simulink model "TIF_avance3"  (R2021b)
settings: Solver=VariableStepAuto  StartTime=0.0  StopTime=10  RelTol=1e-3
undefined symbols (not defined in the file): a11, a13, a23, a31, a33, a42, a44, b, B, J, k1, k10, k11, k2, k3, k4, k5, k6, k7, k8, k9, L1, L2, L3, L4, lamb_ref, Lr, Ls, np, Rpower, Rr, Rs, Rspeed, Rsvolt, TSSimP, Udc
libraries: eeTransforms x2, spsUniversalBridgeLib x1, spsAsynchronousMachineSIUnitsLib x1, spsPWMGeneratorMultilevelLib x1, spsDCVoltageSourceLib x1, spsVoltageMeasurementLib x1, spspowerguiLib x1
settings Model: Creator=Administrador  LastModifiedBy=USER

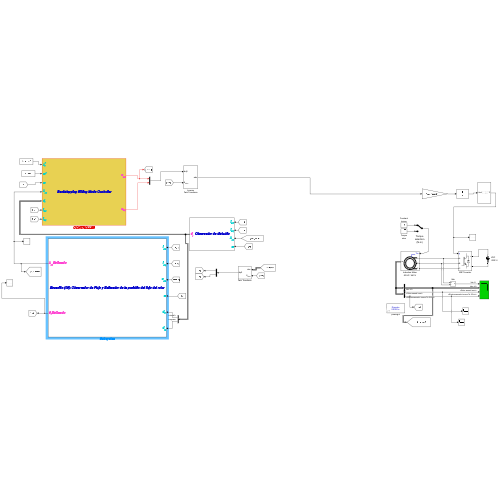
[thumbnail: Simulink's stored preview of the top-level diagram]
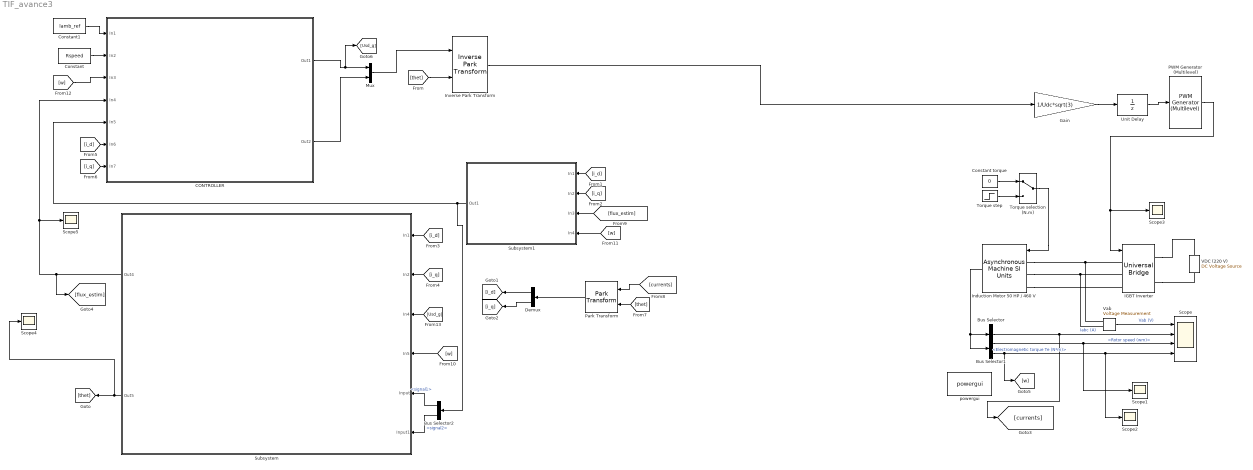
== system TIF_avance3 ==
  Bus Selector : BusSelector  OutputSignals=Stator measurements.Stator current is_a (A),Stator measurements.Stator current is_b (A),Stator measurements.Stator current is_c (A)  OutputAsBus=on
  Bus Selector1 : BusSelector  OutputSignals=Mechanical.Rotor speed (wm),Mechanical.Electromagnetic torque Te (N*m)
  Bus Selector2 : BusSelector  OutputSignals=signal1,signal2
  CONTROLLER : Subsystem
      mask Display:
      | color('magenta'); port_label('output',1,'u_{sd}','texmode', 'on')
      | color('magenta'); port_label('output',2,'u_{sq}','texmode', 'on')
      | color('cyan'); port_label('input',1,'\lambda_r^\ast','texmode', 'on')
      | color('cyan'); port_label('input',2,'\omega^\ast','texmode', 'on')
      | color('cyan'); port_label('input',3,'\omega','texmode', 'on')
      | color('cyan'); port_label('input',4,'\lambda_{rd}','texmode', 'on')
      | color('cyan'); port_label('input',5,'d_{l}','texmode', 'on')
      | color('cyan'); port_label('input',6,'i_{sd}','texmode', 'on')
      | color('cyan'); port_label('input',7,'i_{sq}','texmode', 'on')
      | color('blue'); disp('Backstepping Sliding Mode Controller')
  Constant : Constant  Value=Rspeed
  Constant torque : Constant  Value=0
  Constant1 : Constant  Value=lamb_ref
  Demux : Demux  Outputs=2
  Gain : Gain  Gain=1/Udc*sqrt(3)
  IGBT Inverter : spsUniversalBridgeLib/Universal Bridge  Arms=3  SnubberResistance=1000  SnubberCapacitance=inf  Device=IGBT / Diodes  Ron=1e-3  Lon=0  ForwardVoltages="[  0.8  0.8  ]"  ForwardVoltage=.8  GTOparameters=[ 1e-6 , 1e-6 ]  IGBTparameters=[ 1e-6 , 2e-6 ]  Measurements=None  Measurements_2=None  converterType=Rectifier
      settings: AttributesFormatString=\n
  Induction Motor 50 HP / 460 V : spsAsynchronousMachineSIUnitsLib/Asynchronous Machine SI Units  RotorType=Squirrel-cage  PresetModel=No  MechanicalLoad=Torque Tm  ShowDetailedParameters=on  ReferenceFrame=Stationary  Units=SI  MeasurementBus=off  NominalParameters=[ Rpower, Rsvolt, 60 ]  VoltageRatio=1  Stator=[ Rs Ls ]  Rotor="[ Rr  Lr ]"  Cage1=[ 0.022 0.226/377]  Cage2=[ 0.022 0.226/377]  Lm=Lm  Mechanical="[J  B np ]"  PolePairs=2  InitialConditions="[ 1, 0 ,  0 , 0 , 0 , 0 , 0 , 0 ]"  SimulateSaturation=off  Saturation=[0 0;0 0]  LoadFlowParameters=0  TsPowergui=0  TsBlock=-1  IterativeModel=Trapezoidal non iterative  IterativeDiscreteModel=Trapezoidal non iterative  Pmec=0
      settings: AttributesFormatString=\n
  Inverse Park Transform : eeTransforms/Inverse Park Transform  AxisAlignment=Q-axis  PowerInvariant=off
  Mux : Mux  Inputs=2
  PWM Generator (Multilevel) : spsPWMGeneratorMultilevelLib/PWM Generator (Multilevel)  BridgeType=Half-bridge  NumberOfBridges=3  Fc=10e3  Ts=TSSimP  ShowCarriersOutport=off
      settings: SourceProductBaseCode=PS
  Park Transform : eeTransforms/Park Transform  AxisAlignment=Q-axis  PowerInvariant=off
  Scope : Scope  NumInputPorts=4
  Scope{1..5} (5 alike) : Scope
  Subsystem : Subsystem
      mask Display:
      | color('magenta'); port_label('output',1,'\lambda_{rd}Estimado','texmode', 'on')
      | color('magenta'); port_label('output',2,'\theta_rEstimado','texmode', 'on')
      | color('cyan'); port_label('input',1,'i_{sd}','texmode', 'on')
      | color('cyan'); port_label('input',2,'i_{sq}','texmode', 'on')
      | color('cyan'); port_label('input',3,'u_{sd}','texmode', 'on')
      | color('cyan'); port_label('input',4,' \omega','texmode', 'on')
      | color('cyan'); port_label('input',5,'d_{l1}','texmode', 'on')
      | color('cyan'); port_label('input',6,'d_{l2}','texmode', 'on')
      | 
      | color('blue'); disp('Ecuación (03): Observador de Flujo y Estimador de la posición del flujo del rotor ')
  Subsystem1 : Subsystem
      mask Display:
      | color('magenta'); port_label('output',1,'d_{l}','texmode', 'on')
      | 
      | 
      | color('cyan'); port_label('input',4,'\omega','texmode', 'on')
      | color('cyan'); port_label('input',3,'\lambda_{rd}','texmode', 'on')
      | 
      | color('cyan'); port_label('input',1,'i_{sd}','texmode', 'on')
      | color('cyan'); port_label('input',2,'i_{sq}','texmode', 'on')
      | color('blue'); disp('Observador de disturbio')
  Torque selection (N.m) : ManualSwitch
  Torque step : Step  Time=1.8  After=200  SampleTime=0
  Unit Delay : UnitDelay  SampleTime=TSSimP  HasFrameUpgradeWarning=on
  VDC (220 V) : spsDCVoltageSourceLib/DC Voltage Source  Description=source block  Amplitude=780  Measurements=None
      settings: AttributesFormatString=\n
  Vab : spsVoltageMeasurementLib/Voltage Measurement  Tag=PoWeRsYsTeMmEaSuReMeNt  PhasorSimulation=off  OutputType=Magnitude  PSBequivalent=0
  powergui : spspowerguiLib/powergui  Priority=2  SimulationMode=Discrete  SampleTime=TSSimP  frequency=60  Iterations=50  frequencyindice=60  Pbase=100e6  ErrMax=1e-4  UnitsV=kV  UnitsW=MW  buscounter=0  FunctionMessages=off  echomessages=off  EnableUseOfTLC=off  CurrentSourceSwitches=off  DisableSnubberDevices=off  DisableRonSwitches=off  DisableVfSwitches=off  DisplayEquations=off  AutomaticDiscreteSolvers=off  SolverType=Tustin/Backward Euler (TBE)  Interpol=off  ExternalGateDelay=off  methode=off  Ts=100  x0status=blocks  SPID=off  SwTol=0  HookPort=off  NonlinearTolerance=0  nMaxIteration=15  ContinueOnMaxIteration=off  RestoreLinks=warning  ResistiveCurrentMeasurement=off  Frange=[0:2:500]  Ylog=off  Xlog=on  ShowGrid=off  save=off  variable=ZData  structure=0  ZoomFFT=on  StartTime=0.0  cycles=1  DisplayStyle=off  fundamental=60  FreqAxis=off  MaxFrequency=1000  frequencyindicesteady=1  RmsSteady=1  display=off
  wires:
  Subsystem/1(Out4) -> [flux_estim], CONTROLLER/4(In4), Scope5/1
  Subsystem1/1(Out1) -> Bus Selector2/1, CONTROLLER/5(In5)
  CONTROLLER/1(Out1) -> [Usd_g], Mux/1
  CONTROLLER/2(Out2) -> Mux/2
  Mux/1 -> Inverse Park Transform/1
  Subsystem/2(Out5) -> Scope4/1, [thet]
  [thet] -> Inverse Park Transform/2
  Park Transform/1 -> Demux/1
  Demux/1 -> [i_d]
  Demux/2 -> [i_q]
  [i_q] -> Subsystem1/2(In2)
  [i_d] -> Subsystem1/1(In1)
  [i_q] -> Subsystem/2(In2)
  [i_d] -> Subsystem/1(In1)
  [i_d] -> CONTROLLER/6(In6)
  [i_q] -> CONTROLLER/7(In7)
  [thet] -> Park Transform/2
  PWM Generator (Multilevel)/1 -> Scope3/1, IGBT Inverter/1
  Torque selection (N.m)/1 -> Induction Motor 50 HP / 460 V/1
  Torque step/1 -> Torque selection (N.m)/2
  Bus Selector1/2 -> [w], Scope2/1, Scope/4  "<Electromagnetic torque Te (N*m)>"
  Bus Selector1/1 -> Scope1/1, Scope/3  "<Rotor speed (wm)>"
  Vab/1 -> Scope/1  "Vab (V)"
  Bus Selector/1 -> [currents], Scope/2  "Iabc (A)"
  Gain/1 -> Unit Delay/1
  Unit Delay/1 -> PWM Generator (Multilevel)/1
  Constant torque/1 -> Torque selection (N.m)/1
  Induction Motor 50 HP / 460 V/1 -> Bus Selector1/1, Bus Selector/1
  Inverse Park Transform/1 -> Gain/1
  [currents] -> Park Transform/1
  [flux_estim] -> Subsystem1/3(In3)
  [w] -> Subsystem/4(In5)
  [w] -> Subsystem1/4(In4)
  [w] -> CONTROLLER/3(In3)
  Bus Selector2/1 -> Subsystem/5(Input)  "<signal1>"
  Bus Selector2/2 -> Subsystem/6(Input1)  "<signal2>"
  [Usd_g] -> Subsystem/3(In4)
  Constant/1 -> CONTROLLER/2(In2)
  Constant1/1 -> CONTROLLER/1(In1)
  connections:
  Vab/LConn1 -- Induction Motor 50 HP / 460 V/LConn1 -- IGBT Inverter/LConn1
  Vab/LConn2 -- Induction Motor 50 HP / 460 V/LConn2 -- IGBT Inverter/LConn2
  IGBT Inverter/RConn2 -- VDC (220 V)/LConn1
  IGBT Inverter/RConn1 -- VDC (220 V)/RConn1
  Induction Motor 50 HP / 460 V/LConn3 -- IGBT Inverter/LConn3

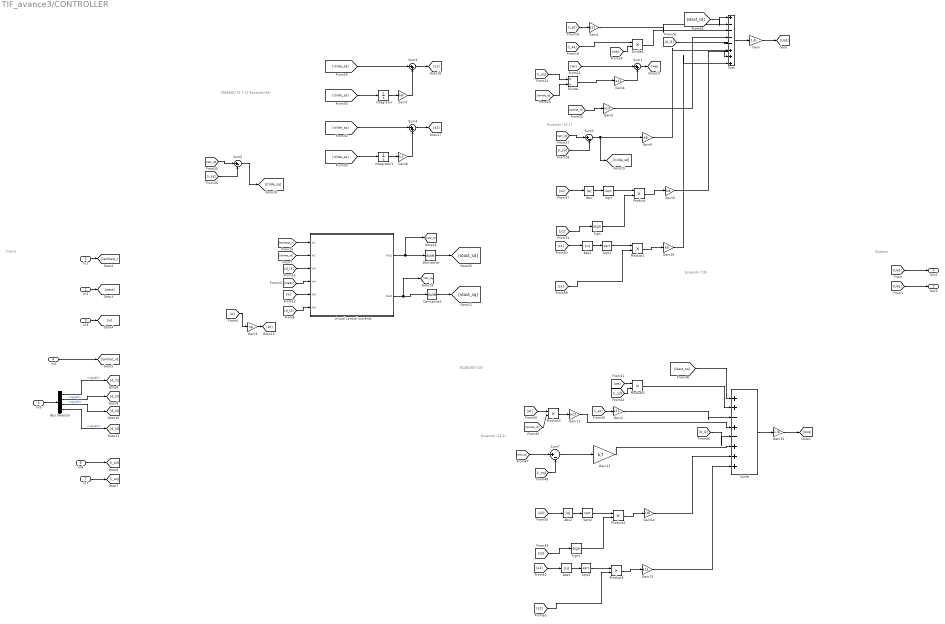
== system TIF_avance3/CONTROLLER ==
  note: ECUACIÓN (20)
  note: Ecuación (15.2)
  note: Ecuación (15.1)
  note: Ecuación (19)
  note: Inputs
  note: Outputs
  note: CREANDO S1 Y S2
      | Ecuación(16)
  In1 : Inport
  In2 : Inport  Port=2
  In3 : Inport  Port=3
  In4 : Inport  Port=4
  In5 : Inport  Port=5
  In6 : Inport  Port=6
  In7 : Inport  Port=7
  Abs{,1..3} (4 alike) : Abs
  Bus Selector : BusSelector  OutputSignals=signal1,signal2,signal3,signal4
  Derivative : Derivative
  Derivative1 : Derivative
  Divide : Product  Inputs=*/
  Divide1 : Product  Inputs=**
  Gain : Gain  Gain=1./b
  Gain1 : Gain  Gain=a11
  Gain10 : Gain  Gain=k9
  Gain11 : Gain  Gain=a23
  Gain12 : Gain  Gain=k7
  Gain13 : Gain  Gain=k11
  Gain14 : Gain  Gain=k10
  Gain15 : Gain  Gain=1./b
  Gain2 : Gain  Gain=a11
  Gain3 : Gain  Gain=np
  Gain4 : Gain  Gain=a31
  Gain5 : Gain  Gain=a13
  Gain6 : Gain  Gain=k6
  Gain7 : Gain  Gain=k6
  Gain8 : Gain  Gain=k7
  Gain9 : Gain  Gain=k8
  Integrator : Integrator
  Integrator1 : Integrator
  Product{,1..5} (6 alike) : Product
  Sign : Signum
  Sign1 : Signum
  Sqrt{,1..3} (4 alike) : Sqrt  SaturateOnIntegerOverflow=on
  Sum : Sum  Inputs=|+|----|+++|
  Sum1 : Sum  Inputs=|++
  Sum2 : Sum  Inputs=|+-
  Sum3 : Sum  Inputs=|++
  Sum4 : Sum  Inputs=|++
  Sum5 : Sum  Inputs=|+-
  Sum6 : Sum  Inputs=|++|-|+|-|+++
  Sum7 : Sum  Inputs=|+-
  "virtual control currents " : Subsystem
      mask Display:
      | color('blue'); port_label('output',1,'i_{sd}^{\ast}','texmode', 'on')
      | color('blue'); port_label('output',2,'i_{sq}^{\ast}','texmode', 'on')
      | color('green'); port_label('input',1,'\lambda_{r}^{\ast}','texmode', 'on')
      | color('green'); port_label('input',2,'\lambda_{rd}','texmode', 'on')
      | color('green'); port_label('input',3,'d_{l3}','texmode', 'on')
      | color('green'); port_label('input',4,'\omega^{\ast}','texmode', 'on')
      | color('green'); port_label('input',5,'\omega','texmode', 'on')
      | color('green'); port_label('input',6,'d_{l4}','texmode', 'on')
      | color('black'); disp(' Ecuación (13)')
  Out1 : Outport
  Out2 : Outport  Port=2
  wires:
  Gain1/1 -> Sum/2
  Sqrt/1 -> Product/1
  In3/1 -> [w]
  In1/1 -> [lambast_r]
  [wr] -> Sum1/1
  "virtual control currents "/2(Out2) -> [iast_sq], Derivative1/1
  [lamhat_rd] -> "virtual control currents "/2(In2)
  [wr] -> Product3/1
  Sum/1 -> Gain/1
  [s1] -> Abs/1
  [lamhat_rd] -> Gain5/1
  [Usq] -> Out2/1
  [itilde_sd] -> Integrator/1
  [w] -> Gain3/1
  Sqrt3/1 -> Product5/1
  In4/1 -> [lamhat_rd]
  Gain4/1 -> Sum1/2
  Integrator1/1 -> Gain8/1
  Abs2/1 -> Sqrt2/1
  [Usd] -> Out1/1
  In2/1 -> [wast]
  Sum6/1 -> Gain15/1
  [d_l4] -> "virtual control currents "/6(In6)
  "virtual control currents "/1(Out1) -> [iast_sd], Derivative/1
  [s2] -> Abs2/1
  Gain/1 -> [Usd]
  [itilde_sq] -> Integrator1/1
  Sum4/1 -> [s2]
  [lambast_r] -> "virtual control currents "/1(In1)
  Gain3/1 -> [wr]
  [s2] -> Abs3/1
  Sum3/1 -> [s1]
  [i_sd] -> Gain1/1
  Abs3/1 -> Sqrt3/1
  [i_sq] -> Divide/1
  Gain14/1 -> Sum6/7
  Divide/1 -> Gain4/1
  Gain13/1 -> Sum6/8
  Product1/1 -> Gain10/1
  [d_l3] -> "virtual control currents "/3(In3)
  [itilde_sq] -> Sum4/1
  Gain5/1 -> Sum/4
  [lamhat_rd] -> Divide/2
  [s1] -> Product1/2
  Sign/1 -> Product/2
  [wast] -> "virtual control currents "/4(In4)
  Product2/1 -> Sum6/2
  Sum1/1 -> [we]
  Derivative1/1 -> [idast_sq]
  Sum2/1 -> Gain6/1, [itilde_sd]
  [w] -> "virtual control currents "/5(In5)
  [d_l1] -> Sum/5
  Integrator/1 -> Gain7/1
  Gain9/1 -> Sum/7
  Gain10/1 -> Sum/8
  Gain8/1 -> Sum4/2
  Gain2/1 -> Sum6/3
  Divide1/1 -> Sum/3
  Product5/1 -> Gain13/1
  [we] -> Divide1/2
  [idast_sq] -> Sum6/1
  [i_sq] -> Divide1/1
  Gain7/1 -> Sum3/2
  [i_sd] -> Sum2/2
  [s2] -> Sign1/1
  Sqrt2/1 -> Product4/1
  Gain15/1 -> [Usq]
  Product4/1 -> Gain14/1
  [s2] -> Product5/2
  Sign1/1 -> Product4/2
  [i_sq] -> Gain2/1
  [lamhat_rd] -> Product3/2
  [itilde_sd] -> Sum3/1
  Gain6/1 -> Sum/6
  Sqrt1/1 -> Product1/1
  Abs/1 -> Sqrt/1
  [idast_sd] -> Sum/1
  Derivative/1 -> [idast_sd]
  [s1] -> Sign/1
  [iast_sq] -> Sum5/1
  [i_sq] -> Sum5/2
  Sum5/1 -> [itilde_sq]
  [we] -> Product2/1
  [iast_sd] -> Sum2/1
  Product/1 -> Gain9/1
  [s1] -> Abs1/1
  Abs1/1 -> Sqrt1/1
  [i_sq] -> Sum7/2
  [i_sd] -> Product2/2
  Gain11/1 -> Sum6/4
  Sum7/1 -> Gain12/1
  Product3/1 -> Gain11/1
  [iast_sq] -> Sum7/1
  Gain12/1 -> Sum6/6
  [d_l2] -> Sum6/5
  In5/1 -> Bus Selector/1
  In7/1 -> [i_sq]
  In6/1 -> [i_sd]
  Bus Selector/1 -> [d_l1]  "<signal1>"
  Bus Selector/2 -> [d_l2]  "<signal2>"
  Bus Selector/3 -> [d_l3]  "<signal3>"
  Bus Selector/4 -> [d_l4]  "<signal4>"

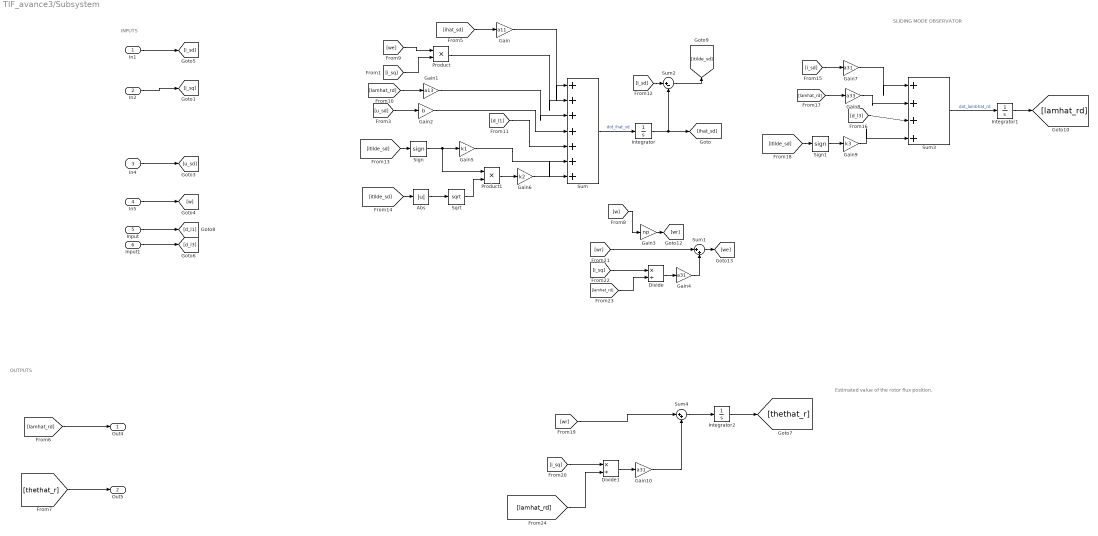
== system TIF_avance3/Subsystem ==
  note: SLIDING MODE OBSERVATOR
  note: OUTPUTS
  note: INPUTS
  note: Estimated value
      | of the rotor flux position.
  In1 : Inport
  In2 : Inport  Port=2
  In4 : Inport  Port=3
  In5 : Inport  Port=4
  Input : Inport  Port=5
  Input1 : Inport  Port=6
  Abs : Abs
  Divide : Product  Inputs=*/
  Divide1 : Product  Inputs=*/
  Gain : Gain  Gain=a11
  Gain1 : Gain  Gain=a13
  Gain10 : Gain  Gain=a31
  Gain2 : Gain  Gain=b
  Gain3 : Gain  Gain=np
  Gain4 : Gain  Gain=a31
  Gain5 : Gain  Gain=k1
  Gain6 : Gain  Gain=k2
  Gain7 : Gain  Gain=a31
  Gain8 : Gain  Gain=a33
  Gain9 : Gain  Gain=k3
  Integrator : Integrator
  Integrator1 : Integrator  InitialCondition=0.2
  Integrator2 : Integrator
  Product : Product
  Product1 : Product
  Sign : Signum
  Sign1 : Signum
  Sqrt : Sqrt  SaturateOnIntegerOverflow=on
  Sum : Sum  Inputs=|+++++++|
  Sum1 : Sum  Inputs=|++
  Sum2 : Sum  Inputs=|+-
  Sum3 : Sum  Inputs=|++++|
  Sum4 : Sum  Inputs=|++
  Out4 : Outport
  Out5 : Outport  Port=2
  wires:
  Input/1 -> [d_l1]
  [w] -> Gain3/1
  Gain4/1 -> Sum1/2
  Gain3/1 -> [wr]
  [lamhat_rd] -> Gain8/1
  Product1/1 -> Gain6/1
  Abs/1 -> Sqrt/1
  Product/1 -> Sum/2
  [i_sd] -> Gain7/1
  [u_sd] -> Gain2/1
  Gain10/1 -> Sum4/2
  [lamhat_rd] -> Out4/1
  Divide1/1 -> Gain10/1
  [i_sq] -> Product/2
  [i_sq] -> Divide1/1
  Gain1/1 -> Sum/3
  Sign/1 -> Product1/1, Gain5/1
  Integrator/1 -> Sum2/2, [ihat_sd]
  [itilde_sd] -> Sign/1
  Gain5/1 -> Sum/6
  In5/1 -> [w]
  Sum/1 -> Integrator/1  "dot_ihat_sd"
  [lamhat_rd] -> Gain1/1
  Integrator1/1 -> [lamhat_rd]
  Sign1/1 -> Gain9/1
  Gain2/1 -> Sum/4
  Sum4/1 -> Integrator2/1
  [lamhat_rd] -> Divide/2
  [wr] -> Sum1/1
  [d_l1] -> Sum/5
  Gain9/1 -> Sum3/4
  In2/1 -> [i_sq]
  [d_l3] -> Sum3/3
  Divide/1 -> Gain4/1
  Gain7/1 -> Sum3/1
  Sum3/1 -> Integrator1/1  "dot_lambhat_rd"
  In4/1 -> [u_sd]
  [wr] -> Sum4/1
  Sqrt/1 -> Product1/2
  Gain/1 -> Sum/1
  [i_sd] -> Sum2/1
  [lamhat_rd] -> Divide1/2
  Input1/1 -> [d_l3]
  [ihat_sd] -> Gain/1
  [thethat_r] -> Out5/1
  [we] -> Product/1
  Integrator2/1 -> [thethat_r]
  In1/1 -> [i_sd]
  Gain8/1 -> Sum3/2
  Sum1/1 -> [we]
  [i_sq] -> Divide/1
  Sum2/1 -> [itilde_sd]
  [itilde_sd] -> Abs/1
  Gain6/1 -> Sum/7
  [itilde_sd] -> Sign1/1

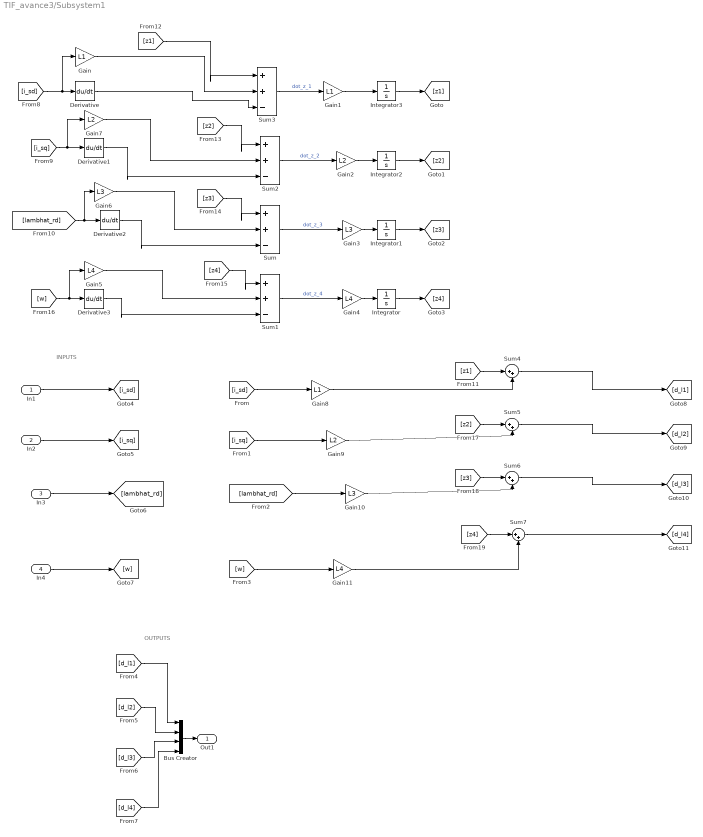
== system TIF_avance3/Subsystem1 ==
  note: OUTPUTS
  note: INPUTS
  In1 : Inport
  In2 : Inport  Port=2
  In3 : Inport  Port=3
  In4 : Inport  Port=4
  Bus Creator : BusCreator  Inputs=4
  Derivative{,1..3} (4 alike) : Derivative
  Gain : Gain  Gain=L1
  Gain1 : Gain  Gain=L1
  Gain10 : Gain  Gain=L3
  Gain11 : Gain  Gain=L4
  Gain2 : Gain  Gain=L2
  Gain3 : Gain  Gain=L3
  Gain4 : Gain  Gain=L4
  Gain5 : Gain  Gain=L4
  Gain6 : Gain  Gain=L3
  Gain7 : Gain  Gain=L2
  Gain8 : Gain  Gain=L1
  Gain9 : Gain  Gain=L2
  Integrator{,1..3} (4 alike) : Integrator
  Sum{,1..3} (4 alike) : Sum  Inputs=|++|-
  Sum{4..7} (4 alike) : Sum  Inputs=|++
  Out1 : Outport
  wires:
  Integrator1/1 -> [z3]
  [i_sd] -> Gain8/1
  Integrator3/1 -> [z1]
  [z3] -> Sum6/1
  Derivative/1 -> Sum3/3
  [z1] -> Sum4/1
  Gain1/1 -> Integrator3/1
  Gain4/1 -> Integrator/1
  Integrator2/1 -> [z2]
  Sum4/1 -> [d_l1]
  Sum7/1 -> [d_l4]
  Sum1/1 -> Gain4/1  "dot_z_4"
  Sum5/1 -> [d_l2]
  Gain10/1 -> Sum6/2
  Gain2/1 -> Integrator2/1
  [z2] -> Sum5/1
  [z2] -> Sum2/1
  Gain9/1 -> Sum5/2
  In4/1 -> [w]
  Sum/1 -> Gain3/1  "dot_z_3"
  Gain8/1 -> Sum4/2
  Gain7/1 -> Sum2/2
  [z4] -> Sum7/1
  Sum2/1 -> Gain2/1  "dot_z_2"
  Integrator/1 -> [z4]
  Gain6/1 -> Sum/2
  Sum3/1 -> Gain1/1  "dot_z_1"
  Gain11/1 -> Sum7/2
  [z1] -> Sum3/1
  In2/1 -> [i_sq]
  [i_sd] -> Gain/1, Derivative/1
  [d_l2] -> Bus Creator/2
  In1/1 -> [i_sd]
  [i_sq] -> Gain7/1, Derivative1/1
  Derivative3/1 -> Sum1/3
  Derivative1/1 -> Sum2/3
  [d_l4] -> Bus Creator/4
  [i_sq] -> Gain9/1
  In3/1 -> [lambhat_rd]
  [w] -> Gain11/1
  [w] -> Gain5/1, Derivative3/1
  [d_l3] -> Bus Creator/3
  [lambhat_rd] -> Gain10/1
  [lambhat_rd] -> Gain6/1, Derivative2/1
  Sum6/1 -> [d_l3]
  [z4] -> Sum1/1
  Gain3/1 -> Integrator1/1
  [z3] -> Sum/1
  Gain/1 -> Sum3/2
  Gain5/1 -> Sum1/2
  Derivative2/1 -> Sum/3
  [d_l1] -> Bus Creator/1
  Bus Creator/1 -> Out1/1

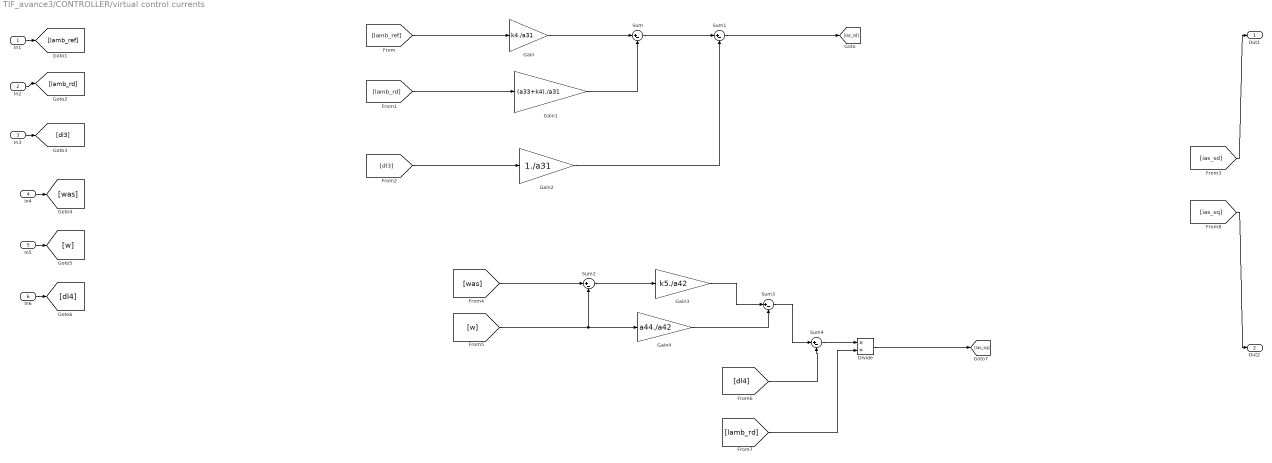
== system TIF_avance3/CONTROLLER/virtual control currents  ==
  In1 : Inport
  In2 : Inport  Port=2
  In3 : Inport  Port=3
  In4 : Inport  Port=4
  In5 : Inport  Port=5
  In6 : Inport  Port=6
  Divide : Product  Inputs=*/  RndMeth=Nearest
  Gain : Gain  Gain=k4./a31
  Gain1 : Gain  Gain=(a33+k4)./a31
  Gain2 : Gain  Gain=1./a31
  Gain3 : Gain  Gain=k5./a42
  Gain4 : Gain  Gain=a44./a42
  Sum{,1..4} (5 alike) : Sum  Inputs=|+-
  Out1 : Outport
  Out2 : Outport  Port=2
  wires:
  In6/1 -> [dl4]
  In4/1 -> [was]
  In3/1 -> [dl3]
  In1/1 -> [lamb_ref]
  Gain4/1 -> Sum3/2
  Gain3/1 -> Sum3/1
  [was] -> Sum2/1
  In2/1 -> [lamb_rd]
  [w] -> Sum2/2, Gain4/1
  [lamb_rd] -> Gain1/1
  Sum2/1 -> Gain3/1
  Gain2/1 -> Sum1/2
  Gain/1 -> Sum/1
  Sum1/1 -> [ias_sd]
  [dl3] -> Gain2/1
  [ias_sd] -> Out1/1
  [lamb_ref] -> Gain/1
  [lamb_rd] -> Divide/2
  [ias_sq] -> Out2/1
  Sum4/1 -> Divide/1
  Divide/1 -> [ias_sq]
  Sum/1 -> Sum1/1
  In5/1 -> [w]
  Sum3/1 -> Sum4/1
  [dl4] -> Sum4/2
  Gain1/1 -> Sum/2
